simulink model "simulation"  (R2025a)
settings: Solver=ode3  StartTime=0.0  StopTime=500  FixedStep=1e-2  RelTol=1e-8  EnableMultiTasking=on
values from neighbouring files (symbols this model uses):
  A = [3.7451e-15 7.6548e-6 0 0;  -4.0887e-6 -6.5527e-2 0 0;  2.3773e-6 5.9026e-4 -0.1426 0;  -8.1593e-14 -5.5355e-2 18.216 0.08333]    [boiler.m]    (also in untitled.m = [ 3.7451e-15    7.6548e-6     0           0)
  A_m = [-0.01 0 0;  0 -0.02 0;  0 0 -0.03]    [boiler.m]    (also in untitled.m = [-0.01   0      0)
  alpha_0 = 8.0314    [boiler.m]    (also in untitled.m)
  alpha_1 = 1.4713    [boiler.m]    (also in untitled.m)
  B = [0.0015 -0.0015 -6.9678e-12;  -5.9548e-5 -9.0316e-5 5.9647e-11;  3.4622e-5 5.2512e-5 3.2492e-11;  -0.0167 0.0239 -1.0733e-9]    [boiler.m]    (also in untitled.m = [ 0.0015       -0.0015       -6.9678e-12)
  B_m = [1 0 0;  0 1 0;  0 0 1]    [boiler.m]    (also in untitled.m = [1 0 0)
  Bound = 1.05e-3    (= 0.00105)    [boiler.m]    (also in untitled.m = 0.001)
  C = [0.05 -0.0484 6.7129 0.05;  0 1 0 0]    [boiler.m]    (also in untitled.m = [ 0.0500       -0.0484        6.7129       0.0500)
  C_m = [0 1 0;  1 0 0]    [boiler.m]    (also in untitled.m = [0 1 0)
  dB = 2.04e-4*[1 2 0;  0 0 0;  1 -1 0;  20 -20 0]    [boiler.m]    (also in untitled.m = dB_fault)
  dC = 0.0002*[1 0 0 0;0 0 0 0]    [boiler.m]    (also in untitled.m = dC_fault)
  fault = 0    [boiler.m]    (also in untitled.m = 1)
  G = [0.968 -114.258 -1;  1     0        0;  0     1        0;  0     0        1]    [boiler.m]    (also in untitled.m = [0.968, -114.258, -1)
  gamma = 0.0013    [boiler.m]    (also in untitled.m)
  Gamma = diag([1.002 0.999 1.001])    [boiler.m]    (also in untitled.m = diag([1,1,1]))
  H = [-0.00264411452837401,  0.276368234354978,  0.00485669922298695;  -0.00212093673792562,  0.126828183853013,  0.00297639139790861;  -11263.6759461726,     221638.898137783,    1282.33499200163]    [boiler.m]    (also in untitled.m = [-0.00264411452837401,  0.276368234354978,   0.0048566992229)
  K_D = [0.0691 0 0 0.0691;  0 0.0691 0 0;  0 0 0.0691 0]    [boiler.m]    (also in untitled.m = [0.0691   0       0       0.0691)
  K_I = 2*[eye(3),[1;0;0]]    [boiler.m]    (also in untitled.m = [2.6355   0       0       2.6355)
  K_P = 0.1*[eye(3),[1;0;0]]    [boiler.m]    (also in untitled.m = [1.3731   0       0       1.3731)
  K_S = 0.01*eye(3)    [boiler.m]    (also in untitled.m = 1.4800*eye(3))
  M = [0.322180266848393,  -23.9048793908242,   -0.198387888997022;  0.273413353570640,  -16.9472760226837,   -0.136907357417107;  1077571.96327408,   -5503793.87571974,   -55561.6496148715]    [boiler.m]    (also in untitled.m = [ 0.322180266848393,   -23.9048793908242,   -0.1983878889970)
  um_factor = 1    [boiler.m]    (also in untitled.m)
settings Model: Creator=Mohmmad Mousavi  LastModifiedBy=Amin
settings SolverCC: AlgebraicLoopSolver=TrustRegion
settings DataIOCC: LimitDataPoints=on  SaveFormat=Array  ReturnWorkspaceOutputs=off
settings OptimizationCC: LifeSpan=inf
settings DebuggingCC: UnconnectedInputMsg=warning  UnconnectedOutputMsg=warning  UnconnectedLineMsg=warning  SFUnexpectedBacktrackingDiag=warning  SFNoUnconditionalDefaultTransitionDiag=warning  SFExecutionAtInitializationDiag=none  ArithmeticOperatorsInVariantConditions=warning
settings HardwareCC: ProdBitPerPointer=32.0  ProdBitPerSizeT=32.0  ProdBitPerPtrDiffT=32.0  ProdLargestAtomicFloat=None  ProdIntDivRoundTo=Undefined  ProdEndianess=Unspecified  ProdWordSize=32.0  ProdHWDeviceType=32-bit Generic
settings ModelReferenceCC: PropagateSignalLabelsOutOfModel=off
settings SFSimCC: SimUseLocalCustomCode=off  CustomCodeUndefinedFunction=UseInterfaceOnly
settings RTWCC: RTWUseLocalCustomCode=off  GPUComputeCapability=3.5
settings CodeAppCC: StateflowObjectComments=on
settings GRTTargetCC: TargetLangStandard=C89/C90 (ANSI)
settings ConfigComp: CovMetricSettings=dw  CovSaveCumulativeToWorkspaceVar=on  CovSaveSingleToWorkspaceVar=on  CovExternalEMLEnable=off

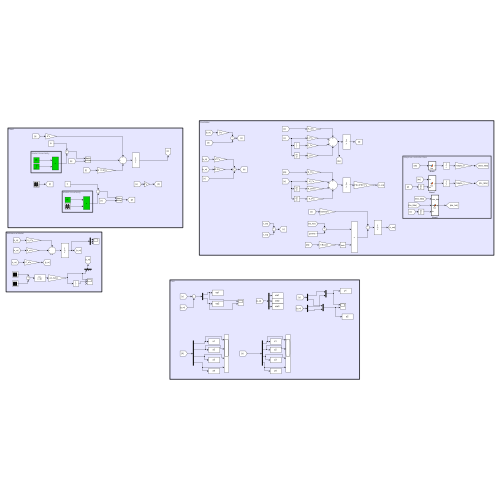
[thumbnail: Simulink's stored preview of the top-level diagram]
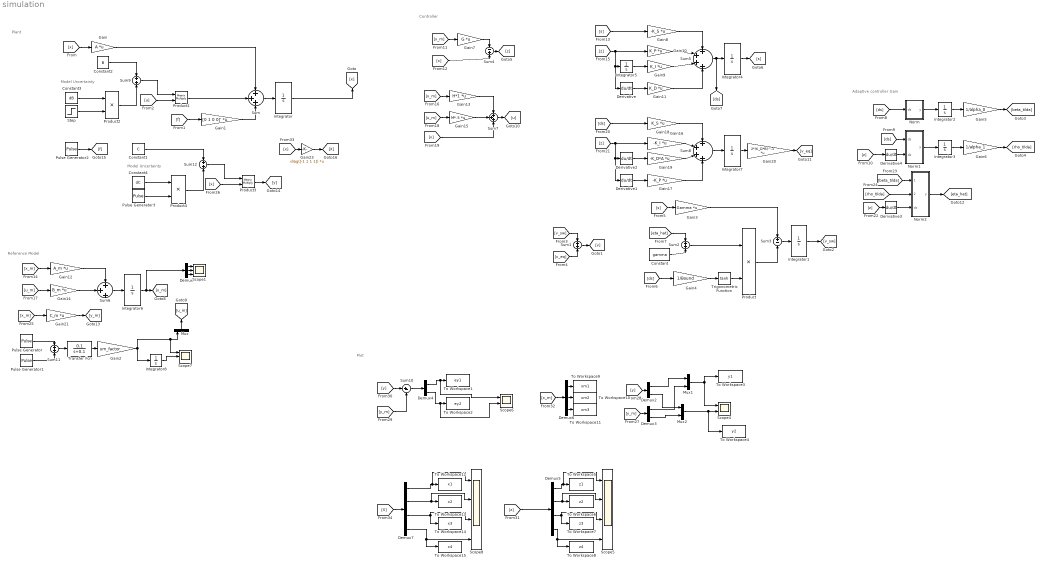
== system simulation ==
  note: Model Uncertainty
  note: Controller
  note: Plot
  note: Adaptive controller Gain
  note: Reference Model
  note: Plant
  note: Model Uncertainty
  Constant : Constant  Value=gamma
  Constant1 : Constant  Value=C
  Constant2 : Constant  Value=B
  Constant3 : Constant  Value=dB
  Constant4 : Constant  Value=dC
  Demux : Demux  Outputs=3
  Demux2 : Demux  Outputs=2
  Demux3 : Demux  Outputs=2
  Demux4 : Demux  Outputs=2
  Demux5 : Demux
  Demux6 : Demux  Outputs=3
  Demux7 : Demux
  Derivative{,1..4} (5 alike) : Derivative
  Gain : Gain  Gain=A  Multiplication=Matrix(K*u)
  Gain1 : Gain  Gain=[0 1 0 0]'  Multiplication=Matrix(K*u)
  Gain10 : Gain  Gain=K_P  Multiplication=Matrix(K*u)
  Gain11 : Gain  Gain=K_D  Multiplication=Matrix(K*u)
  Gain12 : Gain  Gain=A_m  Multiplication=Matrix(K*u)
  Gain13 : Gain  Gain=H*1  Multiplication=Matrix(K*u)
  Gain14 : Gain  Gain=B_m  Multiplication=Matrix(K*u)
  Gain15 : Gain  Gain=M*.5  Multiplication=Matrix(K*u)
  Gain16 : Gain  Gain=-K_I  Multiplication=Matrix(K*u)
  Gain17 : Gain  Gain=-K_P  Multiplication=Matrix(K*u)
  Gain18 : Gain  Gain=K_S  Multiplication=Matrix(K*u)
  Gain19 : Gain  Gain=-K_D*A  Multiplication=Matrix(K*u)
  Gain2 : Gain  Gain=um_factor
  Gain20 : Gain  Gain=2*(K_D*B)^-1  Multiplication=Matrix(K*u)
  Gain21 : Gain  Gain=C_m  Multiplication=Matrix(K*u)
  Gain23 : Gain  Gain=diag([-1 1 1 1])  Multiplication=Matrix(K*u)
  Gain3 : Gain  Gain=Gamma  Multiplication=Matrix(K*u)
  Gain4 : Gain  Gain=1/Bound
  Gain5 : Gain  Gain=1/alpha_0
  Gain6 : Gain  Gain=1/alpha_1
  Gain7 : Gain  Gain=G  Multiplication=Matrix(K*u)
  Gain8 : Gain  Gain=-K_S  Multiplication=Matrix(K*u)
  Gain9 : Gain  Gain=K_I  Multiplication=Matrix(K*u)
  Integrator : Integrator  InitialCondition=[50 60 9 -950]
  Integrator1 : Integrator  InitialCondition=zeros(3,1)
  Integrator{2..5,7} (5 alike) : Integrator
  Integrator6 : Integrator  InitialCondition=[ 60 9 0.05]
  Integrator8 : Integrator  InitialCondition=35
  Mux : Mux  Inputs=3
  Mux1 : Mux  Inputs=2
  Mux2 : Mux  Inputs=2
  Norm : MATLAB Function  TreatAsAtomicUnit=on
  Norm1 : MATLAB Function  TreatAsAtomicUnit=on
  Norm2 : MATLAB Function  TreatAsAtomicUnit=on
  Product : Product
  Product1 : Product  Multiplication=Matrix(*)
  Product2 : Product
  Product3 : Product  Multiplication=Matrix(*)
  Product4 : Product
  Pulse Generator : DiscretePulseGenerator  PulseType=Time based  Amplitude=1.9  Period=100  PulseWidth=50
  Pulse Generator1 : DiscretePulseGenerator  PulseType=Time based  Amplitude=-.5  Period=100  PulseWidth=50  PhaseDelay=50
  Pulse Generator2 : DiscretePulseGenerator  PulseType=Time based  Amplitude=fault  Period=60  PulseWidth=50
  Pulse Generator3 : DiscretePulseGenerator  PulseType=Time based  Period=100  PulseWidth=50
  Scope1 : Scope  NumInputPorts=3
      settings: ActiveDisplayYMinimum=-5  ActiveDisplayYMaximum=5  DataLoggingSaveFormat=Array
  Scope4 : Scope  NumInputPorts=2
      settings: ActiveDisplayYMinimum=-5  ActiveDisplayYMaximum=5  DataLoggingVariableName=ScopeData3  DataLoggingSaveFormat=Array
  Scope5 : Scope  NumInputPorts=4
      settings: ActiveDisplayYMinimum=-5  ActiveDisplayYMaximum=5  DataLoggingVariableName=ScopeData4  DataLoggingSaveFormat=Array
  Scope6 : Scope  NumInputPorts=2
      settings: ActiveDisplayYMinimum=-5  ActiveDisplayYMaximum=5  DataLoggingVariableName=ScopeData5  DataLoggingSaveFormat=Array
  Scope7 : Scope  NumInputPorts=3
      settings: ActiveDisplayYMinimum=-5  ActiveDisplayYMaximum=5  DataLoggingVariableName=ScopeData6  DataLoggingSaveFormat=Array
  Scope8 : Scope  NumInputPorts=4
      settings: ActiveDisplayYMinimum=-5  ActiveDisplayYMaximum=5  DataLoggingVariableName=ScopeData7  DataLoggingSaveFormat=Array
  Step : Step  Time=80  After=1.5  SampleTime=0
  Sum : Sum  Inputs=+++
  Sum{1..2,9,11..12} (5 alike) : Sum
  Sum10 : Sum  Inputs=|+-
  Sum3 : Sum  Inputs=+-
  Sum4 : Sum  Inputs=-+
  Sum5 : Sum  Inputs=++++
  Sum6 : Sum  Inputs=+++
  Sum7 : Sum  Inputs=+++
  Sum8 : Sum  Inputs=++++
  To Workspace1 : ToWorkspace  VariableName=ey1  SaveFormat=Timeseries  SampleTime=-1
  To Workspace10 : ToWorkspace  VariableName=xm2  SaveFormat=Timeseries  SampleTime=-1
  To Workspace11 : ToWorkspace  VariableName=xm3  SaveFormat=Timeseries  SampleTime=-1
  To Workspace12 : ToWorkspace  VariableName=x1  SaveFormat=Timeseries  SampleTime=-1
  To Workspace13 : ToWorkspace  VariableName=x2  SaveFormat=Timeseries  SampleTime=-1
  To Workspace14 : ToWorkspace  VariableName=x3  SaveFormat=Timeseries  SampleTime=-1
  To Workspace15 : ToWorkspace  VariableName=x4  SaveFormat=Timeseries  SampleTime=-1
  To Workspace2 : ToWorkspace  VariableName=ey2  SaveFormat=Timeseries  SampleTime=-1
  To Workspace3 : ToWorkspace  VariableName=y1  SaveFormat=Timeseries  SampleTime=-1
  To Workspace4 : ToWorkspace  VariableName=y2  SaveFormat=Timeseries  SampleTime=-1
  To Workspace5 : ToWorkspace  VariableName=z1  SaveFormat=Timeseries  SampleTime=-1
  To Workspace6 : ToWorkspace  VariableName=z2  SaveFormat=Timeseries  SampleTime=-1
  To Workspace7 : ToWorkspace  VariableName=z3  SaveFormat=Timeseries  SampleTime=-1
  To Workspace8 : ToWorkspace  VariableName=z4  SaveFormat=Timeseries  SampleTime=-1
  To Workspace9 : ToWorkspace  VariableName=xm1  SaveFormat=Timeseries  SampleTime=-1
  Transfer Fcn : TransferFcn  Numerator=[0.1]  Denominator=[1 0.1]
  Trigonometric Function : Trigonometry  Operator=tanh
  wires:
  [x] -> Gain/1
  [f] -> Gain1/1
  [u] -> Product1/2
  Product1/1 -> Sum/2
  Gain/1 -> Sum/1
  Gain1/1 -> Sum/3
  Sum/1 -> Integrator/1
  Sum1/1 -> [v]
  [v_sw] -> Sum1/1
  [v_eq] -> Sum1/2
  [s] -> Gain3/1
  Gain3/1 -> Sum3/1
  Integrator1/1 -> [v_sw]
  [ds] -> Gain4/1
  Constant/1 -> Sum2/2
  Gain4/1 -> Trigonometric Function/1
  Sum2/1 -> Product/1
  Trigonometric Function/1 -> Product/2
  Product/1 -> Sum3/2
  Sum3/1 -> Integrator1/1
  Integrator2/1 -> Gain5/1
  Gain5/1 -> [beta_tilda]
  [ds] -> Norm/1(ds)
  Norm/1(y) -> Integrator2/1
  Integrator3/1 -> Gain6/1
  Gain6/1 -> [rho_tilda]
  [ds] -> Norm1/1(ds)
  Norm1/1(y) -> Integrator3/1
  Sum4/1 -> [z]
  [x] -> Sum4/2
  [x_m] -> Gain7/1
  Gain7/1 -> Sum4/1
  [s] -> Gain8/1
  Integrator5/1 -> Gain9/1
  Gain10/1 -> Sum5/2
  Gain8/1 -> Sum5/1
  Gain9/1 -> Sum5/3
  Sum5/1 -> Integrator4/1, [ds]
  Integrator4/1 -> [s]
  [z] -> Derivative/1, Integrator5/1, Gain10/1
  Derivative/1 -> Gain11/1
  Gain11/1 -> Sum5/4
  [x_m] -> Gain12/1
  [u_m] -> Gain14/1
  Gain14/1 -> Sum6/2
  Gain12/1 -> Sum6/1
  Sum6/1 -> Integrator6/1
  Integrator6/1 -> Demux/1, [x_m]
  Mux/1 -> [u_m]
  [x_m] -> Gain13/1
  [u_m] -> Gain15/1
  Gain13/1 -> Sum7/1
  Gain15/1 -> Sum7/2
  [v] -> Sum7/3
  Sum7/1 -> [u]
  Demux/1 -> Scope1/1
  Demux/2 -> Scope1/2
  Demux/3 -> Scope1/3
  Integrator/1 -> [x]
  [ds] -> Gain18/1
  Derivative2/1 -> Gain19/1
  Gain16/1 -> Sum8/2
  Gain18/1 -> Sum8/1
  Sum8/1 -> Integrator7/1
  [z] -> Derivative2/1, Derivative1/1, Gain16/1
  Derivative1/1 -> Gain17/1
  Gain17/1 -> Sum8/4
  Integrator7/1 -> Gain20/1
  Gain20/1 -> [v_eq]
  Norm2/1(y) -> [eta_hat]
  [beta_tilda] -> Norm2/1(beta_tilda)
  [z] -> Derivative3/1
  Derivative3/1 -> Norm2/3(dz)
  [z] -> Derivative4/1
  Derivative4/1 -> Norm1/2(dz)
  [x_m] -> Gain21/1
  Gain21/1 -> [y_m]
  [y] -> Demux2/1
  [y_m] -> Demux3/1
  Demux2/1 -> Mux1/1
  Demux3/1 -> Mux1/2
  Demux2/2 -> Mux2/1
  Demux3/2 -> Mux2/2
  Mux1/1 -> Scope4/1, To Workspace3/1
  Mux2/1 -> To Workspace4/1, Scope4/2
  Constant2/1 -> Sum9/1
  Constant3/1 -> Product2/1
  Pulse Generator/1 -> Sum11/1
  Product2/1 -> Sum9/2
  Sum9/1 -> Product1/1
  Demux4/1 -> Scope6/1, To Workspace1/1
  Demux4/2 -> Scope6/2, To Workspace2/1
  [y] -> Sum10/1
  [y_m] -> Sum10/2
  Sum10/1 -> Demux4/1
  [z] -> Demux5/1
  Demux5/4 -> Scope5/4, To Workspace8/1
  Demux5/3 -> To Workspace7/1, Scope5/3
  Demux5/1 -> Scope5/1, To Workspace5/1
  Gain19/1 -> Sum8/3
  Integrator8/1 -> Scope7/2
  Pulse Generator1/1 -> Sum11/2
  Gain2/1 -> Integrator8/1, Scope7/1, Mux/1
  Step/1 -> Product2/2
  Pulse Generator2/1 -> [f]
  [eta_hat] -> Sum2/1
  [rho_tilda] -> Norm2/2(rho_tilda)
  [x_m] -> Demux6/1
  Demux6/2 -> To Workspace10/1
  Demux6/1 -> To Workspace9/1
  Demux6/3 -> To Workspace11/1
  Demux5/2 -> Scope5/2, To Workspace6/1
  Demux7/4 -> Scope8/4, To Workspace15/1
  Demux7/3 -> To Workspace14/1, Scope8/3
  Demux7/1 -> Scope8/1, To Workspace12/1
  Demux7/2 -> Scope8/2, To Workspace13/1
  Sum11/1 -> Transfer Fcn/1
  Transfer Fcn/1 -> Gain2/1
  [X] -> Demux7/1
  [x] -> Gain23/1
  Gain23/1 -> [X]
  [x] -> Product3/2
  Product3/1 -> [y]
  Constant1/1 -> Sum12/1
  Constant4/1 -> Product4/1
  Product4/1 -> Sum12/2
  Sum12/1 -> Product3/1
  Pulse Generator3/1 -> Product4/2

== matlab function simulation/Norm ==
  data: ds input; y output
function y = fcn(ds)
%#codegen

y = norm(ds);

== matlab function simulation/Norm2 ==
  data: beta_tilda input; y output; rho_tilda input; dz input
function y = fcn(beta_tilda,rho_tilda,dz)
%#codegen

y = 0*(beta_tilda + rho_tilda*norm(dz));

== matlab function simulation/Norm1 ==
  data: ds input; y output; dz input
function y = fcn(ds,dz)
%#codegen

y = norm(ds)*norm(dz);
